simulink model "model"  (R2019b)
settings: Solver=ode45  StartTime=0.0  StopTime=10  RelTol=1e-3
values from neighbouring files (symbols this model uses):
  K1 = 10    [right_parts.m]    (also in rp_for_check.m)
  K3 = 1    [right_parts.m]    (also in rp_for_check.m)
  K4 = 3    [right_parts.m]    (also in rp_for_check.m)
  Kf = 0.2506628274631    (= 0.250662827463)    [right_parts.m]    (also in rp_for_check.m)
  Klin = 0.11239753    [right_parts.m]    (also in rp_for_check.m)
  T1 = 0.005    [right_parts.m]    (also in rp_for_check.m)
  T3 = 0.05    [right_parts.m]    (also in rp_for_check.m)
  T4 = 0.01    [right_parts.m]    (also in rp_for_check.m)
  Tf = 0.1    [right_parts.m]    (also in rp_for_check.m)
  xi = 0.07    [right_parts.m]    (also in rp_for_check.m)
settings Model: Creator=Roman  LastModifiedBy=Roman

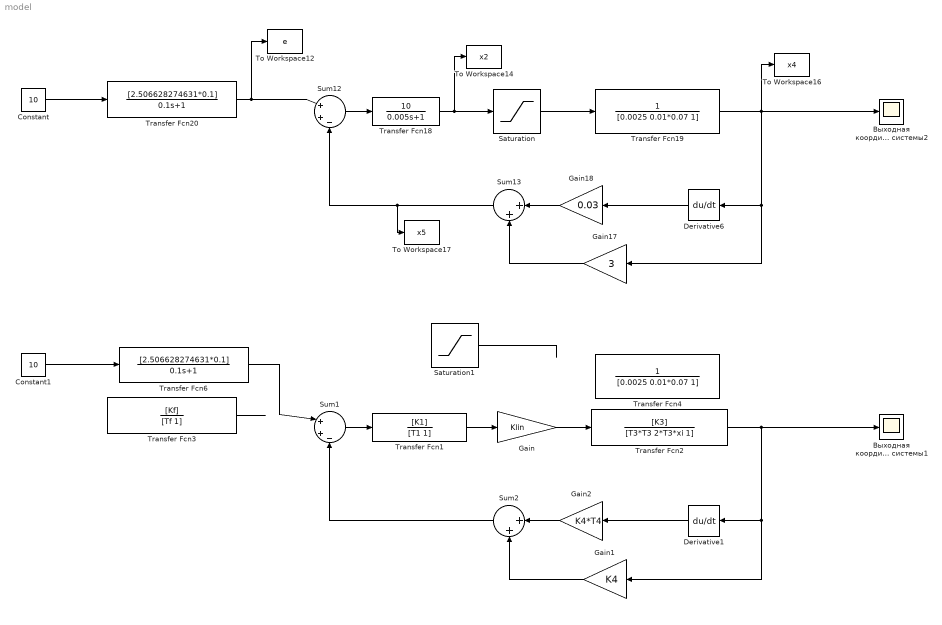
== system model ==
  Constant : Constant  Value=10
  Constant1 : Constant  Value=10
  Derivative1 : Derivative  CoefficientInTFapproximation=1
  Derivative6 : Derivative  CoefficientInTFapproximation=1
  Gain : Gain  Gain=Klin
  Gain1 : Gain  Gain=K4
  Gain17 : Gain  Gain=3
  Gain18 : Gain  Gain=0.03
  Gain2 : Gain  Gain=K4*T4
  Saturation : Saturate  UpperLimit=pi/6  LowerLimit=-pi/6
  Saturation1 : Saturate  UpperLimit=pi/6  LowerLimit=-pi/6
  Sum1 : Sum  Inputs=|++-
  Sum12 : Sum  Inputs=|++-
  Sum13 : Sum  Inputs=|++
  Sum2 : Sum  Inputs=|++
  To Workspace12 : ToWorkspace  VariableName=e  SampleTime=-1
  To Workspace14 : ToWorkspace  VariableName=x2  SampleTime=-1
  To Workspace16 : ToWorkspace  VariableName=x4  SampleTime=-1
  To Workspace17 : ToWorkspace  VariableName=x5  SampleTime=-1
  Transfer Fcn1 : TransferFcn  Numerator=[K1]  Denominator=[T1 1]
  Transfer Fcn18 : TransferFcn  Numerator=[10]  Denominator=[0.005 1]
  Transfer Fcn19 : TransferFcn  Denominator=[0.0025 0.01*0.07 1]
  Transfer Fcn2 : TransferFcn  Numerator=[K3]  Denominator=[T3*T3 2*T3*xi 1]
  Transfer Fcn20 : TransferFcn  Numerator=[2.506628274631*0.1]  Denominator=[0.1 1]
  Transfer Fcn3 : TransferFcn  Numerator=[Kf]  Denominator=[Tf 1]
  Transfer Fcn4 : TransferFcn  Denominator=[0.0025 0.01*0.07 1]
  Transfer Fcn6 : TransferFcn  Numerator=[2.506628274631*0.1]  Denominator=[0.1 1]
  Выходная координата линеаризованной первым способом системы1 : Scope
  Выходная координата линеаризованной первым способом системы2 : Scope
  wires:
  Transfer Fcn19/1 -> Выходная координата линеаризованной первым способом системы2/1, Gain17/1, Derivative6/1, To Workspace16/1
  Saturation/1 -> Transfer Fcn19/1
  Gain17/1 -> Sum13/2
  Derivative6/1 -> Gain18/1
  Sum13/1 -> To Workspace17/1, Sum12/3
  Gain18/1 -> Sum13/1
  Transfer Fcn18/1 -> Saturation/1, To Workspace14/1
  Transfer Fcn20/1 -> To Workspace12/1, Sum12/1
  Constant/1 -> Transfer Fcn20/1
  Sum12/1 -> Transfer Fcn18/1
  Transfer Fcn2/1 -> Выходная координата линеаризованной первым способом системы1/1, Gain1/1, Derivative1/1
  Sum1/1 -> Transfer Fcn1/1
  Transfer Fcn3/1 -> ?
  Constant1/1 -> Transfer Fcn6/1
  Gain/1 -> Transfer Fcn2/1
  Transfer Fcn1/1 -> Gain/1
  Gain2/1 -> Sum2/1
  Sum2/1 -> Sum1/3
  Gain1/1 -> Sum2/2
  Derivative1/1 -> Gain2/1
  Saturation1/1 -> ?
  Transfer Fcn6/1 -> Sum1/1
